simulink model "fft_hdl"  (R2018a)
settings: Solver=VariableStepAuto  StartTime=0.0  StopTime=10.0  RelTol=1e-3
libraries: dspobslib x1
settings Model: Creator=berke  LastModifiedBy=berke

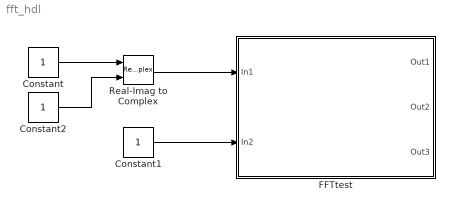
== system fft_hdl ==
  Constant : Constant  OutDataTypeStr=fixdt(1,16,5)  SampleTime=0.1
  Constant1 : Constant  OutDataTypeStr=boolean  SampleTime=0.1
  Constant2 : Constant  OutDataTypeStr=fixdt(1,16,5)  SampleTime=0.1
  FFTtest : Subsystem
  Real-Imag to Complex : RealImagToComplex
  wires:
  Real-Imag to Complex/1 -> FFTtest/1(In1)
  Constant1/1 -> FFTtest/2(In2)
  Constant/1 -> Real-Imag to Complex/1
  Constant2/1 -> Real-Imag to Complex/2

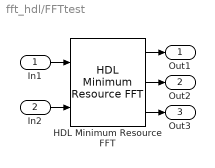
== system fft_hdl/FFTtest ==
  In1 : Inport
  In2 : Inport  Port=2
  HDL Minimum Resource FFT : dspobslib/HDL Minimum Resource FFT  N=16  rnd=Floor  sat=Saturate  sinemode=Same word length as input  sineWL=10  prodmode=Same as input  prodWL=16  prodFL=13  accumode=Same as input  accuWL=18  accuFL=10  outputmode=Same as input  outputWL=16  outputFL=8
      settings: SourceProductName=DSP System Toolbox  SourceProductBaseCode=DS
  Out1 : Outport
  Out2 : Outport  Port=2
  Out3 : Outport  Port=3
  wires:
  HDL Minimum Resource FFT/3 -> Out3/1
  HDL Minimum Resource FFT/1 -> Out1/1
  In2/1 -> HDL Minimum Resource FFT/2
  In1/1 -> HDL Minimum Resource FFT/1
  HDL Minimum Resource FFT/2 -> Out2/1
